simulink model "FOPDT_Tustin"  (R2018b)
settings: Solver=FixedStepDiscrete  StartTime=0.0  StopTime=150  FixedStep=1  RelTol=1e-3
settings Model: Creator=Trips  LastModifiedBy=Trips
settings ConfigComp: PLC_TargetIDE=step7  PLC_GenerateReport=off  PLC_LaunchReport=off

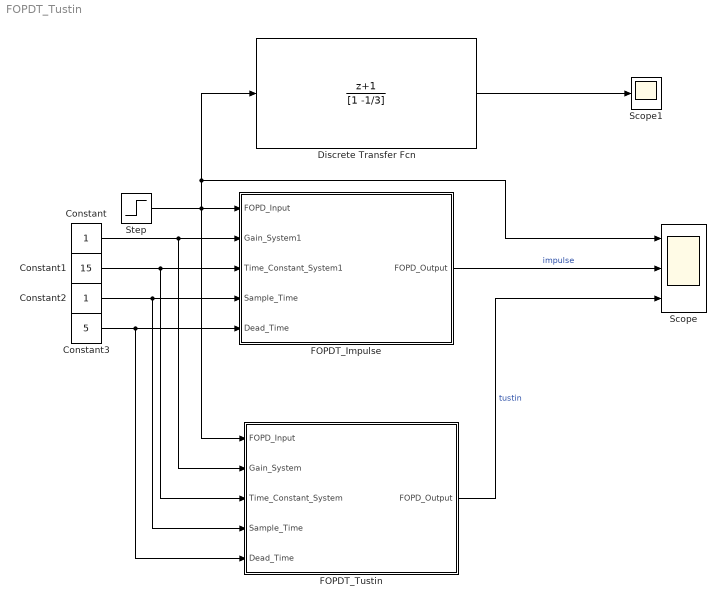
== system FOPDT_Tustin ==
  Constant : Constant
  Constant1 : Constant  Value=15
  Constant2 : Constant
  Constant3 : Constant  Value=5
  Discrete Transfer Fcn : DiscreteTransferFcn  Numerator=[1 1]  Denominator=[1 -1/3]  SampleTime=1  a0EqualsOne=on
  FOPDT_Impulse : Subsystem  TreatAsAtomicUnit=on  SystemSampleTime=1
  FOPDT_Tustin : Subsystem  TreatAsAtomicUnit=on  SystemSampleTime=1
  Scope : Scope  NumInputPorts=3
  Scope1 : Scope
  Step : Step  SampleTime=0
  wires:
  FOPDT_Impulse/1(FOPD_Output) -> Scope/2  "impulse"
  Constant3/1 -> FOPDT_Impulse/5(" Dead_Time"), FOPDT_Tustin/5(" Dead_Time")
  Step/1 -> FOPDT_Tustin/1(FOPD_Input), Scope/1, Discrete Transfer Fcn/1, FOPDT_Impulse/1(FOPD_Input)
  Constant/1 -> FOPDT_Impulse/2(Gain_System1), FOPDT_Tustin/2(Gain_System)
  Constant2/1 -> FOPDT_Impulse/4(Sample_Time), FOPDT_Tustin/4(Sample_Time)
  Constant1/1 -> FOPDT_Impulse/3(Time_Constant_System1), FOPDT_Tustin/3(Time_Constant_System)
  FOPDT_Tustin/1(FOPD_Output) -> Scope/3  "tustin"
  Discrete Transfer Fcn/1 -> Scope1/1

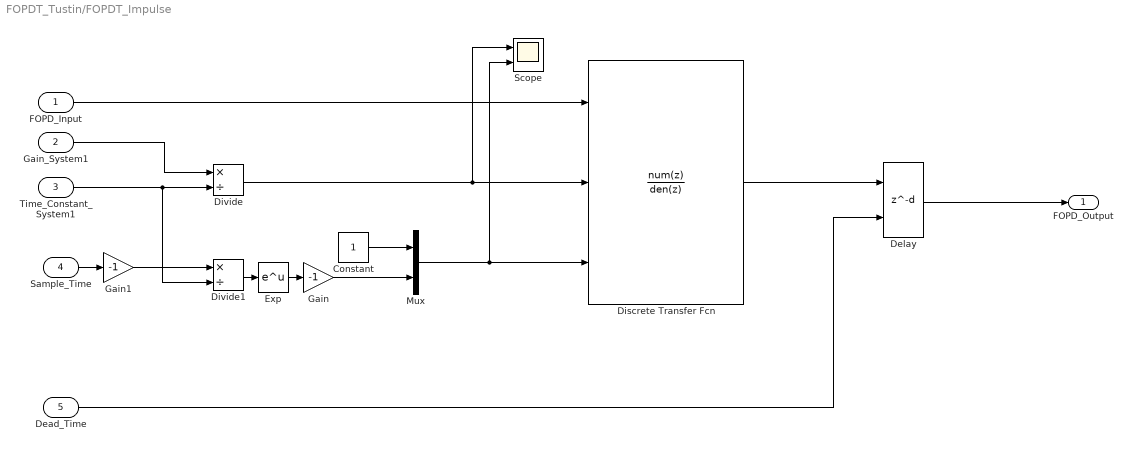
== system FOPDT_Tustin/FOPDT_Impulse ==
  FOPD_Input : Inport
  Gain_System1 : Inport  Port=2
  Time_Constant_System1 : Inport  Port=3
  Sample_Time : Inport  Port=4
  " Dead_Time" : Inport  Port=5
  Constant : Constant
  Delay : Delay  DelayLengthSource=Input port  DelayLength=600  DelayLengthUpperLimit=800
      settings: InputPortMap=u0,p1
  Discrete Transfer Fcn : DiscreteTransferFcn  NumeratorSource=Input port  DenominatorSource=Input port  a0EqualsOne=on
      settings: InputPortMap=u0,p1,p3
  Divide : Product  Inputs=*/
  Divide1 : Product  Inputs=*/
  Exp : Math  SaturateOnIntegerOverflow=on
  Gain : Gain  Gain=-1
  Gain1 : Gain  Gain=-1
  Mux : Mux  Inputs=2
  Scope : Scope  NumInputPorts=2
  FOPD_Output : Outport
  wires:
  Gain1/1 -> Divide1/1
  Time_Constant_System1/1 -> Divide1/2, Divide/2
  FOPD_Input/1 -> Discrete Transfer Fcn/1
  Discrete Transfer Fcn/1 -> Delay/1
  Exp/1 -> Gain/1
  Constant/1 -> Mux/1
  Mux/1 -> Scope/2, Discrete Transfer Fcn/3
  Divide1/1 -> Exp/1
  Gain_System1/1 -> Divide/1
  Gain/1 -> Mux/2
  " Dead_Time"/1 -> Delay/2
  Sample_Time/1 -> Gain1/1
  Divide/1 -> Scope/1, Discrete Transfer Fcn/2
  Delay/1 -> FOPD_Output/1

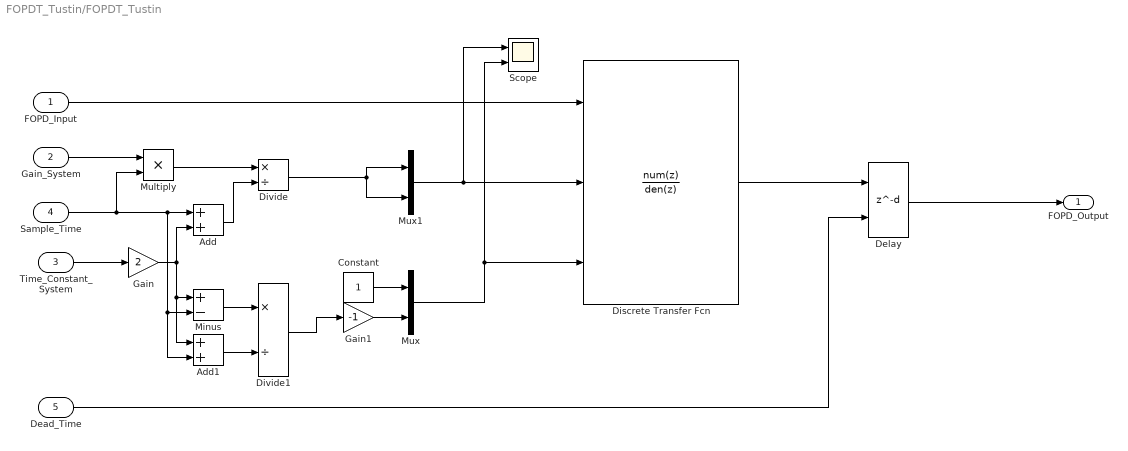
== system FOPDT_Tustin/FOPDT_Tustin ==
  FOPD_Input : Inport
  Gain_System : Inport  Port=2
  Time_Constant_System : Inport  Port=3
  Sample_Time : Inport  Port=4
  " Dead_Time" : Inport  Port=5
  Add : Sum
  Add1 : Sum
  Constant : Constant
  Delay : Delay  DelayLengthSource=Input port  DelayLength=600  DelayLengthUpperLimit=800
      settings: InputPortMap=u0,p1
  Discrete Transfer Fcn : DiscreteTransferFcn  NumeratorSource=Input port  DenominatorSource=Input port  SampleTime=1  a0EqualsOne=on
      settings: InputPortMap=u0,p1,p3
  Divide : Product  Inputs=*/
  Divide1 : Product  Inputs=*/
  Gain : Gain  Gain=2
  Gain1 : Gain  Gain=-1
  Minus : Sum  Inputs=+-
  Multiply : Product
  Mux : Mux  Inputs=2
  Mux1 : Mux  Inputs=2
  Scope : Scope  NumInputPorts=2
  FOPD_Output : Outport
  wires:
  FOPD_Input/1 -> Discrete Transfer Fcn/1
  Discrete Transfer Fcn/1 -> Delay/1
  Mux/1 -> Scope/2, Discrete Transfer Fcn/3
  " Dead_Time"/1 -> Delay/2
  Sample_Time/1 -> Add1/2, Minus/2, Add/1, Multiply/2
  Mux1/1 -> Scope/1, Discrete Transfer Fcn/2
  Time_Constant_System/1 -> Gain/1
  Delay/1 -> FOPD_Output/1
  Gain_System/1 -> Multiply/1
  Multiply/1 -> Divide/1
  Gain/1 -> Add1/1, Minus/1, Add/2
  Add/1 -> Divide/2
  Divide/1 -> Mux1/2, Mux1/1
  Constant/1 -> Mux/1
  Minus/1 -> Divide1/1
  Add1/1 -> Divide1/2
  Divide1/1 -> Gain1/1
  Gain1/1 -> Mux/2
